simulink model "TZ_H1simulink"  (R2019a)
settings: Solver=FixedStepDiscrete  StartTime=0.0  StopTime=10.0  FixedStep=Ts  RelTol=1e-3
libraries: cstblocks x1, simulink x1
settings Model: Creator=3711538  LastModifiedBy=3711538

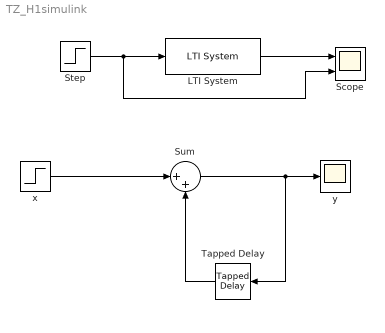
== system TZ_H1simulink ==
  LTI System : cstblocks/LTI System  sys=H1  IC=[]
  Scope : Scope  NumInputPorts=2
  Step : Step  Time=0  SampleTime=0
  Sum : Sum  Inputs=|++
  Tapped Delay : simulink/Discrete/Tapped Delay  vinit=0.0  samptime=Ts  NumDelays=4  DelayOrder=Oldest  includeCurrent=off
  x : Step  SampleTime=0
  y : Scope
  wires:
  Step/1 -> Scope/2, LTI System/1
  x/1 -> Sum/1
  Sum/1 -> Tapped Delay/1, y/1
  Tapped Delay/1 -> Sum/2
  LTI System/1 -> Scope/1
